simulink model "BD_PAR_saber_cosim"  (Simulink 4.1.1)
settings: Solver=ode1  SolverMode=SingleTasking  StartTime=0.0  StopTime=max(cyc_mph(:,1))  FixedStep=1  MaxStep=1  RelTol=1e-3  AbsTol=1e-3
undefined symbols (not defined in the file): cs_charge_deplete_bool, cs_electric_decel_spd, cs_electric_launch_spd_hi, cs_electric_launch_spd_lo, cs_hi_soc, cs_lo_soc, cs_off_trq_frac, cyc_mph, ess_on, ex_calc, fc_emis, fc_map_spd, fc_max_trq, fc_on, fc_spd_scale, fc_trq_scale, fc_tstat, fd_ratio, gb_dnshift_load, gb_dnshift_spd, gb_gears_num, gb_num_init, gb_ratio, gb_shift_delay, gb_upshift_load, gb_upshift_spd, mc_map_spd, mc_max_trq, mc_output_switch, mc_overtrq_factor, mc_spd_scale, mc_trq_scale, tc_mc_to_fc_ratio, time_step, tx_speed_dep, vc_clutch_bool, vc_fc_warm_tmp_frac, vc_idle_bool, vc_idle_spd, vc_launch_spd, wh_radius
libraries: lib_cosimulation x9, lib_outputs x7, lib_controls x6, lib_transmission x4, lib_wheel x2, simulink3 x2, lib_help x2, lib_interactive x1, lib_accessory x1, lib_drive_cycle x1, lib_exhaust x1, lib_fuel_converter x1
(part 1 of 2)
settings Model: LastModifiedBy=ssprik  SaveTime=off  SaveOutput=off  LimitDataPoints=off  UnconnectedLineMsg=none  RTWTemplateMakefile=grt_vc.tmf  ExtModeTrigMode=oneshot  ExtModeArmWhenConnect=off

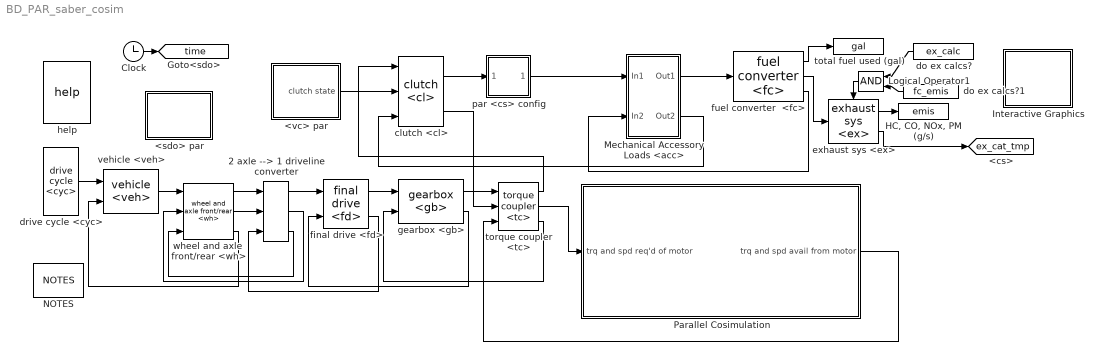
== system BD_PAR_saber_cosim ==
  2 axle --> 1 driveline converter : lib_wheel/2 axle --> 1 driveline converter
      settings: RTWFcnNameOpts=Auto  RTWFileNameOpts=Auto
  <sdo> par : Subsystem
      settings: RTWFcnNameOpts=Auto  RTWFileNameOpts=Auto
      mask Display: image(imread('bdi_sdo.jpg'))
  <vc> par : Subsystem
      settings: RTWFcnNameOpts=Auto  RTWFileNameOpts=Auto
      mask Display: image(imread('bdi_vc.jpg'))
  Clock : Clock
      settings: DisplayTime=off  Decimation=10
  "HC, CO, NOx, PM (g/s)" : ToWorkspace  VariableName=emis  SampleTime=0  SaveFormat=Array
  Interactive Graphics : Subsystem  BlockChoice=off
      link override off/Live Inputs/veh/roll res interactive: BlockChoice=roll res force req (N)
      settings: AttributesFormatString=%<BlockChoice>  TemplateBlock=lib_interactive/Interactive Graphics  MemberBlocks=off,on  RTWFcnNameOpts=Auto  RTWFileNameOpts=Auto
  Logical Operator1 : Logic  Orientation=left  Operator=AND  Inputs=2
  Mechanical Accessory Loads <acc> : Subsystem
      settings: RTWFcnNameOpts=Auto  RTWFileNameOpts=Auto
      mask Display: image(imread('bdi_acc_pic.bmp'))
  NOTES : lib_help/NOTES
  Parallel Cosimulation : Subsystem
      settings: RTWFcnNameOpts=Auto  RTWFileNameOpts=Auto
      mask Display: image(imread('par_cosim.bmp'))
  clutch <cl> : lib_transmission/clutch <cl>  slip_spd=vc_launch_spd  maxtrq=max(fc_max_trq)*fc_trq_scale
  do ex calcs? : Constant  Orientation=left  Value=ex_calc
  do ex calcs?1 : Constant  Orientation=left  Value=fc_emis
  drive cycle <cyc> : lib_drive_cycle/drive cycle <cyc>
  exhaust sys <ex> : lib_exhaust/exhaust sys <ex>
  final drive <fd> : lib_transmission/final drive <fd>
  fuel converter  <fc> : lib_fuel_converter/fuel converter  <fc>
      link override fuel use and EO emis Configurable Subsystem: BlockChoice=fuel use and EO emis
  gearbox <gb> : lib_transmission/gearbox <gb>
  help : lib_help/help
  par <cs> config : Subsystem  BlockChoice=electric assist control strategy <cs>
      settings: AttributesFormatString=%<BlockChoice>  TemplateBlock=lib_controls/par <cs> config  MemberBlocks=Adaptive control strategy <cs>,Fuzzy Logic control strategy <cs>,Fuzzy Logic control strategy with Emissions <cs>,electric assist control strategy <cs>,electric assist control strategy bal <cs>  RTWFcnNameOpts=Auto  RTWFileNameOpts=Auto
  torque coupler <tc> : lib_transmission/torque coupler <tc>
  total fuel used (gal) : ToWorkspace  VariableName=gal  SampleTime=0  SaveFormat=Array
  vehicle <veh> : lib_vehicle/vehicle <veh>
      link override record achieved force outputs/rolling resistance force: BlockChoice=force req'd to overcome rolling resistance (N)
      link override rolling resistance force: BlockChoice=force req'd to overcome rolling resistance (N)
      link override vehicle speed: BlockChoice=vehicle speed (m/s)
  wheel and axle  front/rear <wh> : lib_wheel/wheel and axle  front//rear <wh>
  tag scope: ex_cat_tmp=global, time=global
  wires:
  wheel and axle  front/rear <wh>/3 -> vehicle <veh>/2
  final drive <fd>/2 -> 2 axle --> 1 driveline converter/3
  final drive <fd>/1 -> gearbox <gb>/1
  drive cycle <cyc>/1 -> vehicle <veh>/1
  clutch <cl>/1 -> par <cs> config/1("trq and spd req'd into clutch (N*m, rad/s)")
  fuel converter  <fc>/2 -> exhaust sys <ex>/1
  do ex calcs?/1 -> Logical Operator1/1
  fuel converter  <fc>/1 -> total fuel used (gal)/1
  exhaust sys <ex>/1 -> "HC, CO, NOx, PM (g/s)"/1
  Logical Operator1/1 -> exhaust sys <ex>/Enable
  do ex calcs?1/1 -> Logical Operator1/2
  Clock/1 -> [time]
  gearbox <gb>/2 -> final drive <fd>/2
  torque coupler <tc>/3 -> gearbox <gb>/2
  torque coupler <tc>/1 -> clutch <cl>/1
  clutch <cl>/2 -> torque coupler <tc>/2
  gearbox <gb>/1 -> torque coupler <tc>/1
  <vc> par/1(clutch state) -> clutch <cl>/2
  torque coupler <tc>/2 -> Parallel Cosimulation/1(trq and spd req'd of motor)
  exhaust sys <ex>/2 -> [ex_cat_tmp]
  Parallel Cosimulation/1(trq and spd avail from motor) -> torque coupler <tc>/3
  par <cs> config/1("trq and spd req'd from engine (N*m, rad/s)") -> Mechanical Accessory Loads <acc>/1(In1)
  Mechanical Accessory Loads <acc>/1(Out1) -> fuel converter  <fc>/1
  fuel converter  <fc>/3 -> Mechanical Accessory Loads <acc>/2(In2)
  Mechanical Accessory Loads <acc>/2(Out2) -> clutch <cl>/3
  vehicle <veh>/1 -> wheel and axle  front/rear <wh>/1
  wheel and axle  front/rear <wh>/1 -> 2 axle --> 1 driveline converter/1
  wheel and axle  front/rear <wh>/2 -> 2 axle --> 1 driveline converter/2
  2 axle --> 1 driveline converter/1 -> final drive <fd>/1
  2 axle --> 1 driveline converter/2 -> wheel and axle  front/rear <wh>/2
  2 axle --> 1 driveline converter/3 -> wheel and axle  front/rear <wh>/3

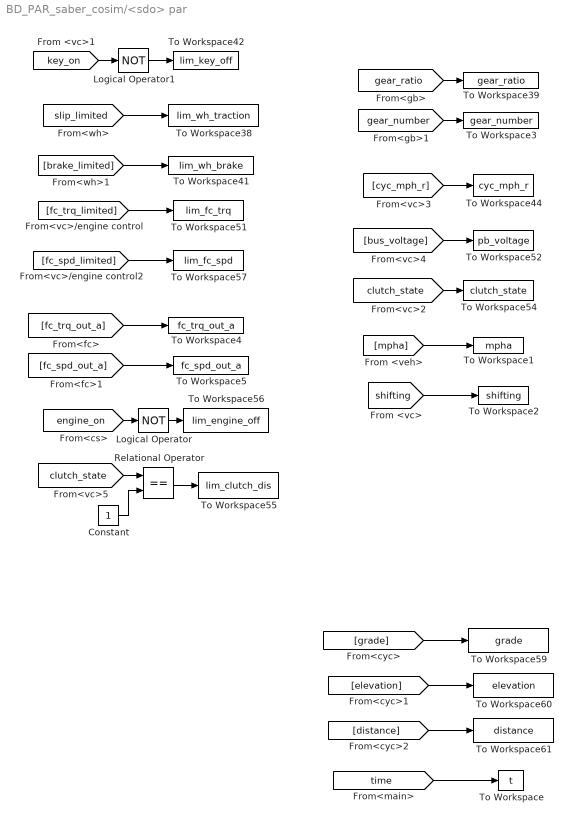
== system BD_PAR_saber_cosim/<sdo> par ==
  Constant : Constant  Value=1
  Logical Operator : Logic  Operator=NOT  Inputs=1
  Logical Operator1 : Logic  Operator=NOT  Inputs=1
  Relational Operator : RelationalOperator  Operator===
  To Workspace : ToWorkspace  VariableName=t  SampleTime=0  SaveFormat=Array
  To Workspace1 : ToWorkspace  VariableName=mpha  SampleTime=-1  SaveFormat=Array
  To Workspace2 : ToWorkspace  VariableName=shifting  SampleTime=-1  SaveFormat=Array
  To Workspace3 : ToWorkspace  VariableName=gear_number  SampleTime=-1  SaveFormat=Array
  To Workspace38 : ToWorkspace  VariableName=lim_wh_traction  SampleTime=-1  SaveFormat=Array
  To Workspace39 : ToWorkspace  VariableName=gear_ratio  SampleTime=-1  SaveFormat=Array
  To Workspace4 : ToWorkspace  VariableName=fc_trq_out_a  SampleTime=-1  SaveFormat=Array
  To Workspace41 : ToWorkspace  VariableName=lim_wh_brake  SampleTime=-1  SaveFormat=Array
  To Workspace42 : ToWorkspace  VariableName=lim_key_off  SampleTime=-1  SaveFormat=Array
  To Workspace44 : ToWorkspace  VariableName=cyc_mph_r  SampleTime=-1  SaveFormat=Array
  To Workspace5 : ToWorkspace  VariableName=fc_spd_out_a  SampleTime=-1  SaveFormat=Array
  To Workspace51 : ToWorkspace  VariableName=lim_fc_trq  SampleTime=-1  SaveFormat=Array
  To Workspace52 : ToWorkspace  VariableName=pb_voltage  SampleTime=-1  SaveFormat=Array
  To Workspace54 : ToWorkspace  VariableName=clutch_state  SampleTime=-1  SaveFormat=Array
  To Workspace55 : ToWorkspace  VariableName=lim_clutch_dis  SampleTime=-1  SaveFormat=Array
  To Workspace56 : ToWorkspace  VariableName=lim_engine_off  SampleTime=-1  SaveFormat=Array
  To Workspace57 : ToWorkspace  VariableName=lim_fc_spd  SampleTime=-1  SaveFormat=Array
  To Workspace59 : ToWorkspace  VariableName=grade  SampleTime=-1  SaveFormat=Array
  To Workspace60 : ToWorkspace  VariableName=elevation  SampleTime=-1  SaveFormat=Array
  To Workspace61 : ToWorkspace  VariableName=distance  SampleTime=-1  SaveFormat=Array
  wires:
  [time] -> To Workspace/1
  [fc_spd_out_a] -> To Workspace5/1
  [fc_trq_out_a] -> To Workspace4/1
  Relational Operator/1 -> To Workspace55/1
  Logical Operator/1 -> To Workspace56/1
  [engine_on] -> Logical Operator/1
  Constant/1 -> Relational Operator/2
  [clutch_state] -> Relational Operator/1
  [distance] -> To Workspace61/1
  [elevation] -> To Workspace60/1
  [grade] -> To Workspace59/1
  [brake_limited] -> To Workspace41/1
  [slip_limited] -> To Workspace38/1
  Logical Operator1/1 -> To Workspace42/1
  [key_on] -> Logical Operator1/1
  [shifting] -> To Workspace2/1
  [mpha] -> To Workspace1/1
  [clutch_state] -> To Workspace54/1
  [bus_voltage] -> To Workspace52/1
  [cyc_mph_r] -> To Workspace44/1
  [gear_ratio] -> To Workspace39/1
  [fc_spd_limited] -> To Workspace57/1
  [fc_trq_limited] -> To Workspace51/1
  [gear_number] -> To Workspace3/1

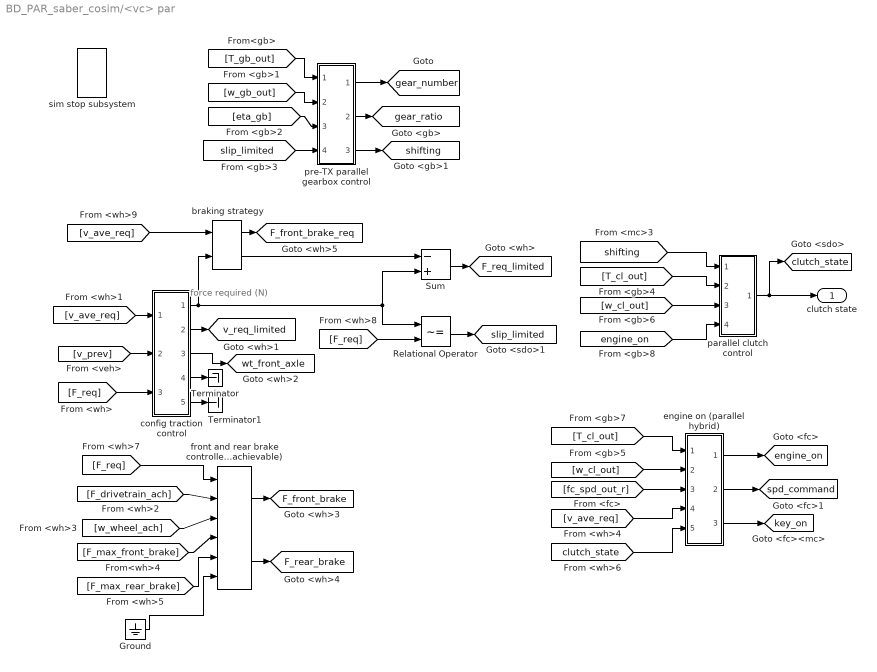
== system BD_PAR_saber_cosim/<vc> par ==
  note: force
      | required (N)
  Ground : Ground
  Relational Operator : RelationalOperator  Operator=~=
  Sum : Sum  Inputs=-+  SaturateOnIntegerOverflow=on
  Terminator : Terminator
  Terminator1 : Terminator
  braking strategy : lib_controls/SubSystem/braking strategy
      settings: RTWFcnNameOpts=Auto  RTWFileNameOpts=Auto
  config traction control : Subsystem  BlockChoice=traction control 2 axle
      settings: AttributesFormatString=%<BlockChoice>  TemplateBlock=lib_controls/SubSystem/config traction control  MemberBlocks=traction control 2 axle,traction control J2452 2 axle  RTWFcnNameOpts=Auto  RTWFileNameOpts=Auto
  engine on (parallel hybrid) : Subsystem
      settings: RTWFcnNameOpts=Auto  RTWFileNameOpts=Auto
  front and rear brake controller (achievable) : lib_controls/SubSystem/front and rear brake controller (achievable)
      settings: RTWFcnNameOpts=Auto  RTWFileNameOpts=Auto
  parallel clutch control : Subsystem
      settings: RTWFcnNameOpts=Auto  RTWFileNameOpts=Auto
  pre-TX parallel gearbox control : Subsystem
      settings: RTWFcnNameOpts=Auto  RTWFileNameOpts=Auto
  sim stop subsystem : lib_controls/SubSystem/sim stop subsystem
      settings: RTWFcnNameOpts=Auto  RTWFileNameOpts=Auto
  clutch state : Outport  Port=1
  tag scope: F_front_brake=global, F_front_brake_req=global, F_rear_brake=global, F_req_limited=global, clutch_state=global, engine_on=global, gear_number=global, gear_ratio=global, key_on=global, shifting=global, slip_limited=global, spd_command=global, v_req_limited=global, wt_front_axle=global
  wires:
  pre-TX parallel gearbox control/3("shifting, out") -> [shifting]
  pre-TX parallel gearbox control/2("gear ratio, out") -> [gear_ratio]
  pre-TX parallel gearbox control/1("gear number, out") -> [gear_number]
  [F_req] -> front and rear brake controller (achievable)/1
  front and rear brake controller (achievable)/2 -> [F_rear_brake]
  [F_max_rear_brake] -> front and rear brake controller (achievable)/5
  [F_max_front_brake] -> front and rear brake controller (achievable)/4
  [w_wheel_ach] -> front and rear brake controller (achievable)/3
  [F_drivetrain_ach] -> front and rear brake controller (achievable)/2
  front and rear brake controller (achievable)/1 -> [F_front_brake]
  [v_ave_req] -> braking strategy/1
  [v_ave_req] -> config traction control/1(time-average vehicle speed  req'd (m/s))
  [F_req] -> Relational Operator/2
  Relational Operator/1 -> [slip_limited]
  parallel clutch control/1(clutch state) -> clutch state/1, [clutch_state]
  [engine_on] -> parallel clutch control/4(engine on)
  [T_cl_out] -> parallel clutch control/2(gb_trq_in_r)
  [w_cl_out] -> parallel clutch control/3(gb_spd_in_r)
  [shifting] -> parallel clutch control/1(shifting)
  Sum/1 -> [F_req_limited]
  [F_req] -> config traction control/3(total tractive force req'd (N))
  config traction control/2(req'd speed (m/s)) -> [v_req_limited]
  [v_prev] -> config traction control/2(vehicle speed at beginning of time  step (m/s))
  braking strategy/1 -> [F_front_brake_req]
  config traction control/1(req'd force (N)) -> Relational Operator/1, Sum/2, braking strategy/2
  braking strategy/2 -> Sum/1
  [clutch_state] -> engine on (parallel hybrid)/5(clutch state)
  engine on (parallel hybrid)/1(engine on) -> [engine_on]
  [T_cl_out] -> engine on (parallel hybrid)/1(trq req'd out of clutch (N*m))
  [w_cl_out] -> engine on (parallel hybrid)/2(spd req'd out of clutch (N*m)1)
  [v_ave_req] -> engine on (parallel hybrid)/4(v_ave_req)
  engine on (parallel hybrid)/2(spd command  (rad/s)) -> [spd_command]
  [fc_spd_out_r] -> engine on (parallel hybrid)/3(fc_spd_out_r)
  engine on (parallel hybrid)/3(key on) -> [key_on]
  [eta_gb] -> pre-TX parallel gearbox control/3(prev. Pout/Pin)
  [w_gb_out] -> pre-TX parallel gearbox control/2(gb_spd_out_r)
  [T_gb_out] -> pre-TX parallel gearbox control/1(gb_trq_out_r)
  [slip_limited] -> pre-TX parallel gearbox control/4(tires are at traction limit)
  config traction control/3(weight on front axle (N)) -> [wt_front_axle]
  config traction control/4(weight on rear axle (N)) -> Terminator/1
  config traction control/5(front/total  traction ratio) -> Terminator1/1
  Ground/1 -> front and rear brake controller (achievable)/6

== system BD_PAR_saber_cosim/Interactive Graphics ==
  off : lib_interactive/off  Tag=Altia_off  Orientation=up

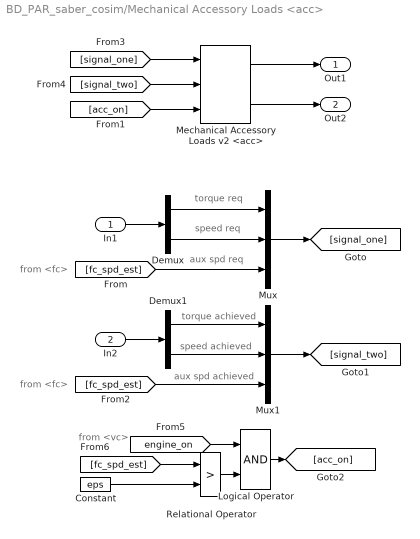
== system BD_PAR_saber_cosim/Mechanical Accessory Loads <acc> ==
  note: from <vc>
  note: aux spd achieved
  note: speed achieved
  note: torque achieved
  note: aux spd req
  note: speed req
  note: torque req
  note: from <fc>
  note: from <fc>
  In1 : Inport  Port=1  LatchInput=off
  In2 : Inport  Port=2  LatchInput=off
  Constant : Constant  Value=eps
  Demux : Demux  Outputs=2  BusSelectionMode=off
  Demux1 : Demux  Outputs=2  BusSelectionMode=off
  Logical Operator : Logic  Operator=AND  Inputs=2
  Mechanical Accessory Loads v2 <acc> : lib_accessory/Mechanical Accessory Loads v2 <acc>  load_on=not(ess_on)*1  acc_max_spd=inf  acc_min_spd=(vc_idle_spd*vc_idle_bool)+eps  ic_mech_trq=0  ic_mech_pwr=0
      link override backward model/mechanical accessories (Nm): BlockChoice=Mechanical Accessories: Speed Dependant and Variable Electrical
      link override estimated mechanical torque/mechanical accessories (Nm): BlockChoice=Mechanical Accessories: Const Mech Var Elect
  Mux : Mux  Inputs=3
  Mux1 : Mux  Inputs=3
  Relational Operator : RelationalOperator  Operator=>
  Out1 : Outport  Port=1
  Out2 : Outport  Port=2
  wires:
  Logical Operator/1 -> [acc_on]
  Relational Operator/1 -> Logical Operator/2
  [engine_on] -> Logical Operator/1
  Constant/1 -> Relational Operator/2
  [fc_spd_est] -> Relational Operator/1
  [fc_spd_est] -> Mux1/3
  Demux1/2 -> Mux1/2
  Demux1/1 -> Mux1/1
  In2/1 -> Demux1/1
  Mux1/1 -> [signal_two]
  [fc_spd_est] -> Mux/3
  Demux/2 -> Mux/2
  Demux/1 -> Mux/1
  In1/1 -> Demux/1
  Mux/1 -> [signal_one]
  [acc_on] -> Mechanical Accessory Loads v2 <acc>/3
  [signal_two] -> Mechanical Accessory Loads v2 <acc>/2
  Mechanical Accessory Loads v2 <acc>/2 -> Out2/1
  Mechanical Accessory Loads v2 <acc>/1 -> Out1/1
  [signal_one] -> Mechanical Accessory Loads v2 <acc>/1

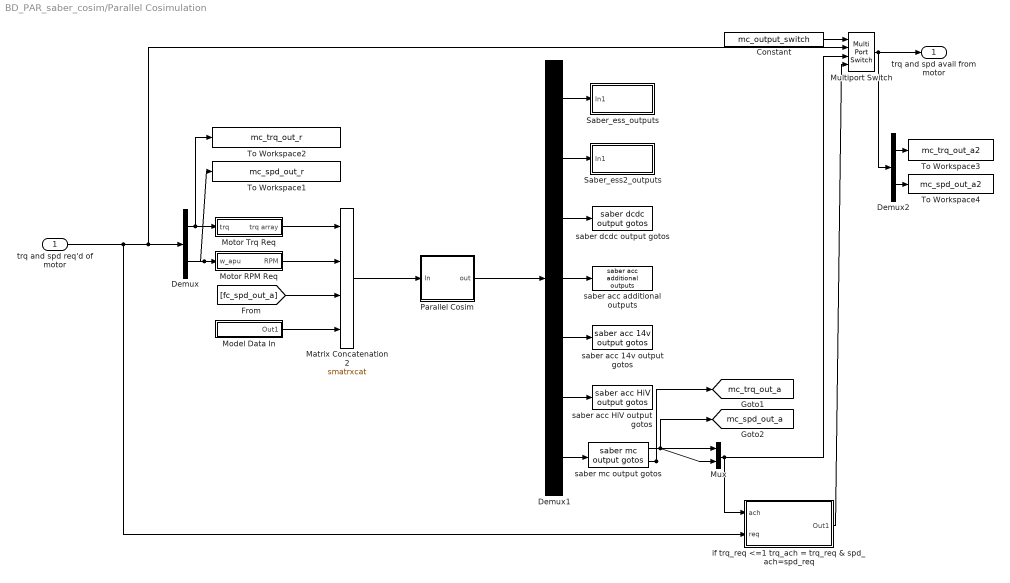
== system BD_PAR_saber_cosim/Parallel Cosimulation ==
  trq and spd req'd of motor : Inport  Port=1  LatchInput=off
  Constant : Constant  Value=mc_output_switch
  Demux : Demux  Outputs=2  BusSelectionMode=off
  Demux1 : Demux  Outputs=[4 4 2 2 30 12 4]  BusSelectionMode=off
  Demux2 : Demux  Outputs=2  BusSelectionMode=off
  Matrix Concatenation2 : S-Function  FunctionName=smatrxcat  Parameters=numInports,catMethod  PortCounts=[]  SFunctionModules=''  mask(Matrix Concatenation){numInports=4, catMethod=Horizontal}
      mask prompts: numInports "Number of inputs:"; catMethod "Concatenation method:"
      mask help: Perform horizontal or vertical concatenation. 1-D vector input signals are treated as column vectors, i.e., [Mx1] matrices. The output is always a matrix.
      mask init:
      | xy = matrxcatmask('icon');
      mask StyleString: edit,popup(Horizontal|Vertical)
      mask Display:
      | plot(xy.x,xy.y);
      | text(0.15,0.86,xy.label);
  Model Data In : Subsystem
      settings: RTWFcnNameOpts=Auto  RTWFileNameOpts=Auto
      mask Display: disp('Parallel')
  Motor RPM Req : Subsystem
      settings: RTWFcnNameOpts=Auto  RTWFileNameOpts=Auto
  Motor Trq Req : Subsystem
      settings: RTWFcnNameOpts=Auto  RTWFileNameOpts=Auto
  Multiport Switch : MultiPortSwitch  Inputs=3
  Mux : Mux  Inputs=2
  Parallel Cosim : Subsystem  BlockChoice=Par Saber Text File Exchange
      settings: AttributesFormatString=%<BlockChoice>  TemplateBlock=lib_cosimulation/Parallel Cosim  MemberBlocks=Par Saber Text File Exchange  RTWFcnNameOpts=Auto  RTWFileNameOpts=Auto
  Saber_ess2_outputs : Subsystem  BlockChoice=Saber_pb2
      settings: AttributesFormatString=%<BlockChoice>  TemplateBlock=lib_outputs/Saber_ess2_outputs  MemberBlocks=Saber_pb2,Saber_rint2  RTWFcnNameOpts=Auto  RTWFileNameOpts=Auto
  Saber_ess_outputs : Subsystem  BlockChoice=Saber_pb
      settings: AttributesFormatString=%<BlockChoice>  TemplateBlock=lib_outputs/Saber_ess_outputs  MemberBlocks=Saber_pb,Saber_rint  RTWFcnNameOpts=Auto  RTWFileNameOpts=Auto
  To Workspace1 : ToWorkspace  VariableName=mc_spd_out_r  SampleTime=-1  SaveFormat=Array
  To Workspace2 : ToWorkspace  VariableName=mc_trq_out_r  SampleTime=-1  SaveFormat=Array
  To Workspace3 : ToWorkspace  VariableName=mc_trq_out_a2  SampleTime=-1  SaveFormat=Array
  To Workspace4 : ToWorkspace  VariableName=mc_spd_out_a2  SampleTime=-1  SaveFormat=Array
  if trq_req <=1 trq_ach = trq_req & spd_ach=spd_req : Subsystem
      settings: RTWFcnNameOpts=Auto  RTWFileNameOpts=Auto
  saber acc 14v output gotos : lib_outputs/saber acc 14v output gotos
      settings: RTWFcnNameOpts=Auto  RTWFileNameOpts=Auto
  saber acc HiV output gotos : lib_outputs/saber acc HiV output gotos
      settings: RTWFcnNameOpts=Auto  RTWFileNameOpts=Auto
  saber acc additional outputs : lib_outputs/saber acc additional outputs
      settings: RTWFcnNameOpts=Auto  RTWFileNameOpts=Auto
  saber dcdc output gotos : lib_outputs/saber dcdc output gotos
      settings: RTWFcnNameOpts=Auto  RTWFileNameOpts=Auto
  saber mc output gotos : lib_outputs/saber mc output gotos
      settings: RTWFcnNameOpts=Auto  RTWFileNameOpts=Auto
  trq and spd avail from motor : Outport  Port=1
  tag scope: mc_spd_out_a=global, mc_trq_out_a=global
  wires:
  trq and spd req'd of motor/1 -> if trq_req <=1 trq_ach = trq_req & spd_ach=spd_req/2(req), Demux/1, Multiport Switch/2
  Matrix Concatenation2/1 -> Parallel Cosim/1(In)
  Demux/1 -> To Workspace2/1, Motor Trq Req/1(trq)
  Demux/2 -> To Workspace1/1, Motor RPM Req/1(w_apu)
  Motor Trq Req/1(trq array) -> Matrix Concatenation2/1
  Motor RPM Req/1(RPM) -> Matrix Concatenation2/2
  Parallel Cosim/1(out) -> Demux1/1
  Demux1/3 -> saber dcdc output gotos/1
  saber mc output gotos/2 -> [mc_trq_out_a], Mux/1
  Demux1/2 -> Saber_ess2_outputs/1(In1)
  Demux1/1 -> Saber_ess_outputs/1(In1)
  saber mc output gotos/1 -> Mux/2, [mc_spd_out_a]
  [fc_spd_out_a] -> Matrix Concatenation2/3
  Model Data In/1(Out1) -> Matrix Concatenation2/4
  Mux/1 -> if trq_req <=1 trq_ach = trq_req & spd_ach=spd_req/1(ach), Multiport Switch/3
  Demux2/1 -> To Workspace3/1
  Demux2/2 -> To Workspace4/1
  Multiport Switch/1 -> trq and spd avail from motor/1, Demux2/1
  Constant/1 -> Multiport Switch/1
  if trq_req <=1 trq_ach = trq_req & spd_ach=spd_req/1(Out1) -> Multiport Switch/4
  Demux1/5 -> saber acc 14v output gotos/1
  Demux1/6 -> saber acc HiV output gotos/1
  Demux1/7 -> saber mc output gotos/1
  Demux1/4 -> saber acc additional outputs/1

== system BD_PAR_saber_cosim/par <cs> config ==
  "trq and spd req'd into clutch (N*m, rad/s)" : Inport  Port=1  LatchInput=off
  electric assist control strategy <cs> : lib_controls/electric assist control strategy <cs>
  "trq and spd req'd from engine (N*m, rad/s)" : Outport  Port=1
  wires:
  "trq and spd req'd into clutch (N*m, rad/s)"/1 -> electric assist control strategy <cs>/1
  electric assist control strategy <cs>/1 -> "trq and spd req'd from engine (N*m, rad/s)"/1

== system BD_PAR_saber_cosim/<vc> par/config traction control ==
  time-average vehicle speed  req'd (m/s) : Inport  Port=1  LatchInput=off
  vehicle speed at beginning of time  step (m/s) : Inport  Port=2  LatchInput=off
  total tractive force req'd (N) : Inport  Port=3  LatchInput=off
  traction control 2 axle : lib_controls/SubSystem/traction control 2 axle
      settings: RTWFcnNameOpts=Auto  RTWFileNameOpts=Auto
  req'd force (N) : Outport  Port=1
  req'd speed (m/s) : Outport  Port=2
  weight on front axle (N) : Outport  Port=3
  weight on rear axle (N) : Outport  Port=4
  front/total  traction ratio : Outport  Port=5
  wires:
  time-average vehicle speed  req'd (m/s)/1 -> traction control 2 axle/1
  vehicle speed at beginning of time  step (m/s)/1 -> traction control 2 axle/2
  total tractive force req'd (N)/1 -> traction control 2 axle/3
  traction control 2 axle/1 -> req'd force (N)/1
  traction control 2 axle/2 -> req'd speed (m/s)/1
  traction control 2 axle/3 -> weight on front axle (N)/1
  traction control 2 axle/4 -> weight on rear axle (N)/1
  traction control 2 axle/5 -> front/total  traction ratio/1

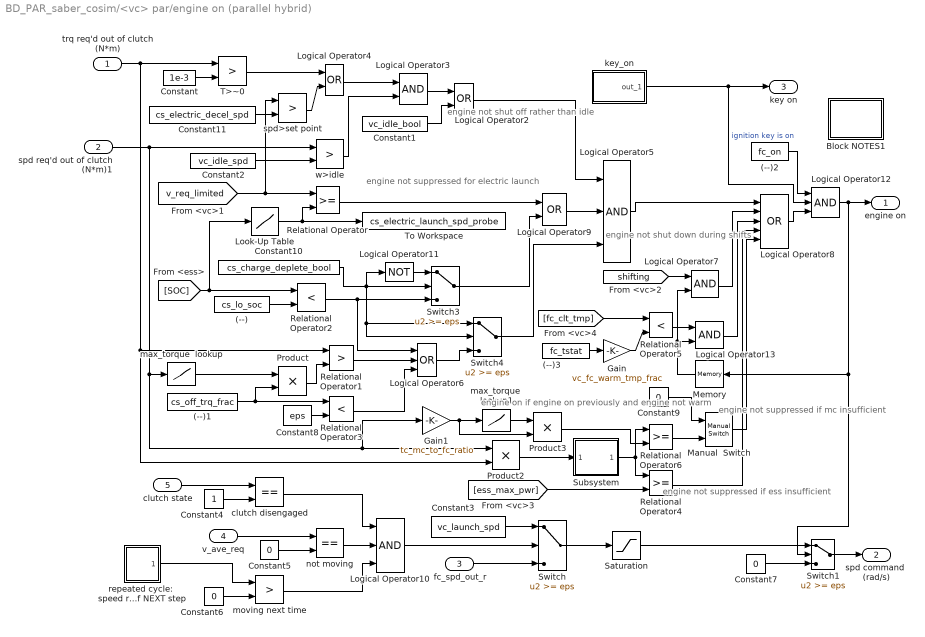
== system BD_PAR_saber_cosim/<vc> par/engine on (parallel hybrid) ==
  note: engine not suppressed
      | if mc insufficient
  note: engine not shut
      | down during shifts
  note: engine on if engine on
      | previously and engine
      | not warm
  note: engine not shut off
      |  rather than idle
  note: engine not
      | suppressed for
      | electric launch
  note: engine not suppressed if
      | ess insufficient
  trq req'd out of clutch (N*m) : Inport  Port=1  LatchInput=off
  spd req'd out of clutch (N*m)1 : Inport  Port=2  LatchInput=off
  fc_spd_out_r : Inport  Port=3  LatchInput=off
  v_ave_req : Inport  Port=4  LatchInput=off
  clutch state : Inport  Port=5  LatchInput=off
  (--) : Constant  Value=cs_lo_soc
  (--)1 : Constant  Value=cs_off_trq_frac
  (--)2 : Constant  Value=fc_on
  (--)3 : Constant  Value=fc_tstat
  Block NOTES1 : Subsystem
      settings: RTWFcnNameOpts=Auto  RTWFileNameOpts=Auto
      mask Display: disp('Block\nNOTES')
  Constant : Constant  Value=1e-3
  Constant1 : Constant  Value=vc_idle_bool
  Constant10 : Constant  Value=cs_charge_deplete_bool
  Constant11 : Constant  Value=cs_electric_decel_spd
  Constant2 : Constant  Value=vc_idle_spd
  Constant3 : Constant  Value=vc_launch_spd
  Constant4 : Constant  Value=1
  Constant{5..7,9} (4 alike) : Constant  Value=0
  Constant8 : Constant  Value=eps
  Gain : Gain  Gain=vc_fc_warm_tmp_frac  Multiplication=Element-wise(K.*u)  SaturateOnIntegerOverflow=on
  Gain1 : Gain  Gain=tc_mc_to_fc_ratio  Multiplication=Element-wise(K.*u)  SaturateOnIntegerOverflow=on
  Logical Operator10 : Logic  Operator=AND  Inputs=3
  Logical Operator11 : Logic  Operator=NOT  Inputs=1
  Logical Operator12 : Logic  Operator=AND  Inputs=3
  Logical Operator13 : Logic  Operator=AND  Inputs=2
  Logical Operator2 : Logic  Operator=OR  Inputs=2
  Logical Operator3 : Logic  Operator=AND  Inputs=2
  Logical Operator4 : Logic  Operator=OR  Inputs=2
  Logical Operator5 : Logic  Operator=AND  Inputs=3
  Logical Operator6 : Logic  Operator=OR  Inputs=3
  Logical Operator7 : Logic  Operator=AND  Inputs=2
  Logical Operator8 : Logic  Operator=OR  Inputs=5
  Logical Operator9 : Logic  Operator=OR  Inputs=2
  Look-Up Table : Lookup  InputValues=[cs_lo_soc cs_hi_soc cs_hi_soc+eps]  OutputValues=[cs_electric_launch_spd_lo cs_electric_launch_spd_hi cs_electric_launch_spd_hi]
  Manual  Switch : simulink3/Nonlinear/Manual Switch  sw=1  action=0
  Memory : Memory  Orientation=left  X0=cyc_mph(1,2)>0  InheritSampleTime=off
      settings: RTWStateStorageClass=Auto
  Product : Product  Inputs=2  Multiplication=Element-wise(.*)  SaturateOnIntegerOverflow=on
  Product2 : Product  Inputs=2  Multiplication=Element-wise(.*)  SaturateOnIntegerOverflow=on
  Product3 : Product  Inputs=2  Multiplication=Element-wise(.*)  SaturateOnIntegerOverflow=on
  Relational Operator : RelationalOperator  Operator=>=
  Relational Operator1 : RelationalOperator  Operator=>
  Relational Operator2 : RelationalOperator  Operator=<
  Relational Operator3 : RelationalOperator  Operator=<
  Relational Operator4 : RelationalOperator  Operator=>=
  Relational Operator5 : RelationalOperator  Operator=<
  Relational Operator6 : RelationalOperator  Operator=>=
  Saturation : Saturate  UpperLimit=max(fc_map_spd)*fc_spd_scale  LowerLimit=vc_idle_spd*vc_idle_bool  LinearizeAsGain=on
  Subsystem : Subsystem  mask(Running Average){n=3}
      mask prompts: n "Averaging Time Steps (#)"
      mask help: Running Average
      settings: RTWFcnNameOpts=Auto  RTWFileNameOpts=Auto
      mask Help: Output is the average of the last (Averaging Time) seconds of input.
      mask Display: disp('Running\nAverage')
  Switch{,1,3..4} (4 alike) : Switch  Threshold=eps
  T>~0 : RelationalOperator  Operator=>
  To Workspace : ToWorkspace  VariableName=cs_electric_launch_spd_probe  SampleTime=-1  SaveFormat=Array
  clutch disengaged : RelationalOperator  Operator===
  key_on : Subsystem  mask(Repeating table){@1=vc_key_on(:,1), @2=vc_key_on(:,2)}
      mask prompts: @1 "Time values:"; @2 "Output values:"
      mask help:
      | Repeating table.
      | Enter values of time and output for first cycle.
      mask init:
      | period = max(@1); t = @1; y = @2;
      settings: RTWFcnNameOpts=Auto  RTWFileNameOpts=Auto
      mask Help: Repeats cycle given in table. Time values should be monotonically increasing.
  max_torque  lookup : Lookup  InputValues=fc_map_spd*fc_spd_scale  OutputValues=fc_max_trq*fc_trq_scale
  max_torque  lookup1 : Lookup  InputValues=mc_map_spd*mc_spd_scale  OutputValues=mc_max_trq*mc_trq_scale*mc_overtrq_factor
  moving next time : RelationalOperator  Operator=>
  not moving : RelationalOperator  Operator===
  repeated cycle:  speed required at end of NEXT step : Subsystem  mask(Forward looking repeating table){t=cyc_mph(:,1), y=cyc_mph(:,2)}
      mask prompts: t "Time values:"; y "Output values:"
      mask help:
      | Forward looking repeating table.
      | Enter values of time and output for first cycle.
      mask init:
      | period = max(t);
      settings: RTWFcnNameOpts=Auto  RTWFileNameOpts=Auto
      mask Help: Repeats cycle given in table with a one time step forward offset. Time values should be monotonically increasing.
  spd>set point : RelationalOperator  Operator=>
  w>idle : RelationalOperator  Operator=>
  engine on : Outport  Port=1
  spd command  (rad/s) : Outport  Port=2
  key on : Outport  Port=3
  wires:
  Subsystem/1(out_1) -> Relational Operator6/1, Relational Operator4/1
  Product3/1 -> Relational Operator6/2
  [ess_max_pwr] -> Relational Operator4/2
  [v_req_limited] -> spd>set point/1, Relational Operator/1
  T>~0/1 -> Logical Operator4/1
  Logical Operator4/1 -> Logical Operator3/1
  spd>set point/1 -> Logical Operator4/2
  Constant11/1 -> spd>set point/2
  spd req'd out of clutch (N*m)1/1 -> w>idle/1, Gain1/1, Product2/1, max_torque  lookup/1
  w>idle/1 -> Logical Operator3/2
  Constant2/1 -> w>idle/2
  Constant9/1 -> Manual  Switch/1
  Manual  Switch/1 -> Logical Operator8/5
  Relational Operator6/1 -> Manual  Switch/2
  Gain1/1 -> Product3/2, max_torque  lookup1/1
  max_torque  lookup1/1 -> Product3/1
  Relational Operator3/1 -> Logical Operator6/3
  Product2/1 -> Subsystem/1(in_1)
  Constant4/1 -> clutch disengaged/2
  clutch state/1 -> clutch disengaged/1
  Constant5/1 -> not moving/2
  v_ave_req/1 -> not moving/1
  not moving/1 -> Logical Operator10/2
  moving next time/1 -> Logical Operator10/3
  clutch disengaged/1 -> Logical Operator10/1
  Constant6/1 -> moving next time/2
  repeated cycle:  speed required at end of NEXT step/1(out_1) -> moving next time/1
  Constant7/1 -> Switch1/3
  Switch1/1 -> spd command  (rad/s)/1
  Saturation/1 -> Switch1/1
  fc_spd_out_r/1 -> Switch/3
  Logical Operator10/1 -> Switch/2
  Switch/1 -> Saturation/1
  Constant3/1 -> Switch/1
  Relational Operator4/1 -> Logical Operator8/4
  (--)/1 -> Relational Operator2/2
  [SOC] -> Look-Up Table/1, Relational Operator2/1
  Logical Operator11/1 -> Switch3/1
  Relational Operator2/1 -> Logical Operator6/1, Switch3/3
  Constant10/1 -> Logical Operator11/1, Switch3/2, Switch4/2, Switch4/1
  Look-Up Table/1 -> To Workspace/1, Relational Operator/2
  Relational Operator/1 -> Logical Operator9/1
  Switch4/1 -> Logical Operator5/3
  Logical Operator9/1 -> Logical Operator5/2
  Logical Operator2/1 -> Logical Operator5/1
  key_on/1(out_1) -> Logical Operator12/2, key on/1  "ignition key is on"
  Logical Operator8/1 -> Logical Operator12/3
  (--)3/1 -> Gain/1
  Gain/1 -> Relational Operator5/2
  Logical Operator13/1 -> Logical Operator8/3
  [fc_clt_tmp] -> Relational Operator5/1
  Relational Operator5/1 -> Logical Operator13/1
  Memory/1 -> Logical Operator13/2, Logical Operator7/2
  Relational Operator1/1 -> Logical Operator6/2
  Logical Operator5/1 -> Logical Operator8/1
  Logical Operator3/1 -> Logical Operator2/1
  Constant1/1 -> Logical Operator2/2
  trq req'd out of clutch (N*m)/1 -> Relational Operator1/1, Product2/2, T>~0/1
  Logical Operator7/1 -> Logical Operator8/2
  [shifting] -> Logical Operator7/1
  Constant/1 -> T>~0/2
  Switch3/1 -> Logical Operator9/2
  Logical Operator6/1 -> Switch4/3
  Constant8/1 -> Relational Operator3/2
  (--)1/1 -> Relational Operator3/1, Product/2
  Product/1 -> Relational Operator1/2
  max_torque  lookup/1 -> Product/1
  (--)2/1 -> Logical Operator12/1
  Logical Operator12/1 -> engine on/1, Memory/1, Switch1/2

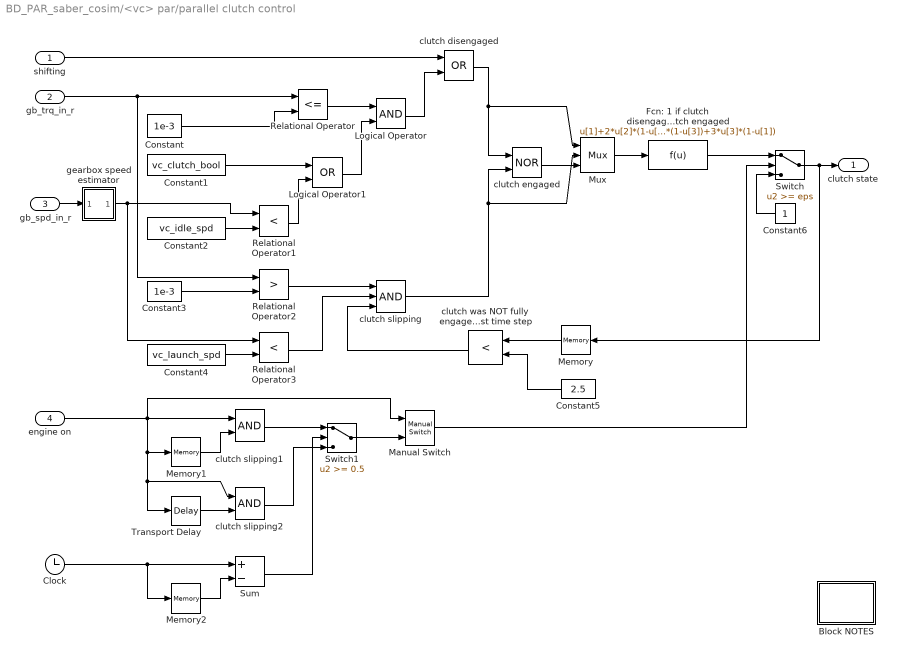
== system BD_PAR_saber_cosim/<vc> par/parallel clutch control ==
  shifting : Inport  Port=1  LatchInput=off
  gb_trq_in_r : Inport  Port=2  LatchInput=off
  gb_spd_in_r : Inport  Port=3  LatchInput=off
  engine on : Inport  Port=4  LatchInput=off
  Block NOTES : Subsystem
      settings: RTWFcnNameOpts=Auto  RTWFileNameOpts=Auto
      mask Display: disp('Block\nNOTES')
  Clock : Clock
      settings: DisplayTime=off  Decimation=10
  Constant : Constant  Value=1e-3
  Constant1 : Constant  Value=vc_clutch_bool
  Constant2 : Constant  Value=vc_idle_spd
  Constant3 : Constant  Value=1e-3
  Constant4 : Constant  Value=vc_launch_spd
  Constant5 : Constant  Orientation=left  Value=2.5
  Constant6 : Constant  Orientation=left  Value=1
  Fcn: 1 if clutch disengaged 2 if clutch slipping 3 if clutch engaged : Fcn  Expr=u[1]+2*u[2]*(1-u[1])*(1-u[3])+3*u[3]*(1-u[1])
  Logical Operator : Logic  Operator=AND  Inputs=2
  Logical Operator1 : Logic  Operator=OR  Inputs=2
  Manual Switch : simulink3/Nonlinear/Manual Switch  sw=1  action=0
  Memory : Memory  Orientation=left  X0=1+(2*(cyc_mph(1,2)>0))  InheritSampleTime=off
      settings: RTWStateStorageClass=Auto
  Memory1 : Memory  X0=cyc_mph(1,2)>0  InheritSampleTime=off
      settings: RTWStateStorageClass=Auto
  Memory2 : Memory  X0=-1  InheritSampleTime=off
      settings: RTWStateStorageClass=Auto
  Mux : Mux  Inputs=3
      settings: DisplayOption=none
  Relational Operator : RelationalOperator  Operator=<=
  Relational Operator1 : RelationalOperator  Operator=<
  Relational Operator2 : RelationalOperator  Operator=>
  Relational Operator3 : RelationalOperator  Operator=<
  Sum : Sum  Inputs=+-  SaturateOnIntegerOverflow=on
  Switch : Switch  Threshold=eps
  Switch1 : Switch  Threshold=0.5
  Transport Delay : TransportDelay  DelayTime=0.2  InitialInput=0  BufferSize=1024  PadeOrder=0
  clutch disengaged : Logic  Operator=OR  Inputs=2
  clutch engaged : Logic  Operator=NOR  Inputs=2
  clutch slipping : Logic  Operator=AND  Inputs=3
  clutch slipping1 : Logic  Operator=AND  Inputs=2
  clutch slipping2 : Logic  Operator=AND  Inputs=2
  clutch was NOT fully engaged during last time step : RelationalOperator  Orientation=left  Operator=<
  gearbox speed estimator : Subsystem
      settings: RTWFcnNameOpts=Auto  RTWFileNameOpts=Auto
  clutch state : Outport  Port=1
  wires:
  Switch/1 -> Memory/1, clutch state/1
  Fcn: 1 if clutch disengaged 2 if clutch slipping 3 if clutch engaged/1 -> Switch/1
  Manual Switch/1 -> Switch/2
  Switch1/1 -> Manual Switch/2
  gearbox speed estimator/1(Out1) -> Relational Operator3/1, Relational Operator1/1
  gb_spd_in_r/1 -> gearbox speed estimator/1(gb_spd_in_r if no gear change)
  Sum/1 -> Switch1/2
  Memory2/1 -> Sum/2
  Clock/1 -> Memory2/1, Sum/1
  clutch slipping2/1 -> Switch1/3
  Transport Delay/1 -> clutch slipping2/2
  clutch slipping1/1 -> Switch1/1
  Memory1/1 -> clutch slipping1/2
  engine on/1 -> Manual Switch/1, clutch slipping2/1, Transport Delay/1, Memory1/1, clutch slipping1/1
  Relational Operator1/1 -> Logical Operator1/2
  Constant2/1 -> Relational Operator1/2
  Mux/1 -> Fcn: 1 if clutch disengaged 2 if clutch slipping 3 if clutch engaged/1
  clutch engaged/1 -> Mux/3
  clutch disengaged/1 -> clutch engaged/1, Mux/1
  Constant3/1 -> Relational Operator2/2
  Relational Operator2/1 -> clutch slipping/1
  clutch slipping/1 -> clutch engaged/2, Mux/2
  Constant4/1 -> Relational Operator3/2
  Relational Operator3/1 -> clutch slipping/2
  Memory/1 -> clutch was NOT fully engaged during last time step/1
  Constant5/1 -> clutch was NOT fully engaged during last time step/2
  clutch was NOT fully engaged during last time step/1 -> clutch slipping/3
  Constant1/1 -> Logical Operator1/1
  Constant/1 -> Relational Operator/2
  Relational Operator/1 -> Logical Operator/1
  Logical Operator1/1 -> Logical Operator/2
  gb_trq_in_r/1 -> Relational Operator2/1, Relational Operator/1
  Logical Operator/1 -> clutch disengaged/2
  shifting/1 -> clutch disengaged/1
  Constant6/1 -> Switch/3

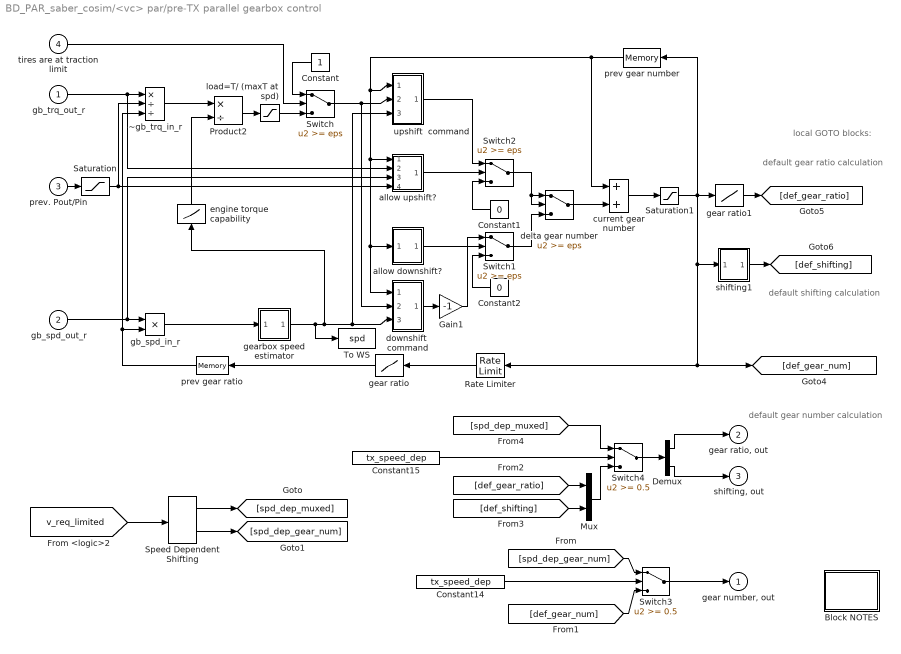
== system BD_PAR_saber_cosim/<vc> par/pre-TX parallel gearbox control ==
  note: local GOTO blocks:
  note: default gear ratio
      | calculation
  note: default shifting
      | calculation
  note: default gear number
      | calculation
  gb_trq_out_r : Inport  Port=1  LatchInput=off
  gb_spd_out_r : Inport  Port=2  LatchInput=off
  prev. Pout/Pin : Inport  Port=3  LatchInput=off
  tires are at traction limit : Inport  Port=4  LatchInput=off
  Block NOTES : Subsystem
      settings: RTWFcnNameOpts=Auto  RTWFileNameOpts=Auto
      mask Display: disp('Block\nNOTES')
  Constant : Constant  Orientation=left  Value=1
  Constant1 : Constant  Orientation=left  Value=0
  Constant14 : Constant  Value=tx_speed_dep
  Constant15 : Constant  Value=tx_speed_dep
  Constant2 : Constant  Orientation=left  Value=0
  Demux : Demux  Outputs=2  BusSelectionMode=off
  Gain1 : Gain  Gain=-1  Multiplication=Element-wise(K.*u)  SaturateOnIntegerOverflow=on
  Mux : Mux  Inputs=2
  Product2 : Product  Inputs=*/  Multiplication=Element-wise(.*)  SaturateOnIntegerOverflow=on
  Rate Limiter : RateLimiter  Orientation=left  RisingSlewLimit=1/(gb_shift_delay+eps)  FallingSlewLimit=-1/(gb_shift_delay+eps)
  Saturation : Saturate  UpperLimit=1  LowerLimit=0.2  LinearizeAsGain=on
  Saturation1 : Saturate  UpperLimit=gb_gears_num  LowerLimit=1  LinearizeAsGain=on
  Speed Dependent Shifting : lib_controls/SubSystem/Speed Dependent Shifting
      settings: RTWFcnNameOpts=Auto  RTWFileNameOpts=Auto
  Switch : Switch  Threshold=eps
  Switch1 : Switch  Threshold=eps
  Switch2 : Switch  Threshold=eps
  Switch3 : Switch  Threshold=0.5
  Switch4 : Switch  Threshold=0.5
  To WS : ToWorkspace  VariableName=spd  SampleTime=-1  SaveFormat=Array
  allow downshift? : Subsystem
      settings: RTWFcnNameOpts=Auto  RTWFileNameOpts=Auto
  allow upshift? : Subsystem
      settings: RTWFcnNameOpts=Auto  RTWFileNameOpts=Auto
  current gear number : Sum  Inputs=++  SaturateOnIntegerOverflow=on
  delta gear number : Switch  Threshold=eps
  downshift  command : Subsystem
      settings: RTWFcnNameOpts=Auto  RTWFileNameOpts=Auto
  engine torque capability : Lookup  Orientation=up  InputValues=fc_map_spd*fc_spd_scale  OutputValues=fc_max_trq*fc_trq_scale+eps
  gb_spd_in_r : Product  Inputs=2  Multiplication=Element-wise(.*)  SaturateOnIntegerOverflow=on
  gear ratio : Lookup  Orientation=left  InputValues=[1:length(gb_ratio)]  OutputValues=gb_ratio
  gear ratio1 : Lookup  InputValues=[1:length(gb_ratio)]  OutputValues=gb_ratio
  gearbox speed estimator : Subsystem
      settings: RTWFcnNameOpts=Auto  RTWFileNameOpts=Auto
  load=T/ (maxT at spd) : Saturate  UpperLimit=1  LowerLimit=0  LinearizeAsGain=on
  prev gear number : Memory  Orientation=left  X0=gb_num_init  InheritSampleTime=off
      settings: RTWStateStorageClass=Auto
  prev gear ratio : Memory  Orientation=left  X0=gb_ratio(gb_num_init)  InheritSampleTime=off
      settings: RTWStateStorageClass=Auto
  shifting1 : Subsystem
      settings: RTWFcnNameOpts=Auto  RTWFileNameOpts=Auto
  upshift  command : Subsystem
      settings: RTWFcnNameOpts=Auto  RTWFileNameOpts=Auto
  ~gb_trq_in_r : Product  Inputs=*//  Multiplication=Element-wise(.*)  SaturateOnIntegerOverflow=on
  "gear number, out" : Outport  Port=1  InitialOutput=0
  "gear ratio, out" : Outport  Port=2  InitialOutput=0
  "shifting, out" : Outport  Port=3  InitialOutput=0
  wires:
  Switch3/1 -> "gear number, out"/1
  Demux/2 -> "shifting, out"/1
  Demux/1 -> "gear ratio, out"/1
  Speed Dependent Shifting/2 -> [spd_dep_gear_num]
  Speed Dependent Shifting/1 -> [spd_dep_muxed]
  [v_req_limited] -> Speed Dependent Shifting/1
  [spd_dep_gear_num] -> Switch3/1
  Switch4/1 -> Demux/1
  [def_shifting] -> Mux/2
  [def_gear_ratio] -> Mux/1
  Mux/1 -> Switch4/3
  [spd_dep_muxed] -> Switch4/1
  Constant15/1 -> Switch4/2
  [def_gear_num] -> Switch3/3
  Constant14/1 -> Switch3/2
  gearbox speed estimator/1(Out1) -> To WS/1, downshift  command/3(engine speed), upshift  command/3(engine speed), engine torque capability/1
  allow upshift?/1(allow shift) -> Switch2/2
  upshift  command/1(command) -> Switch2/1
  Switch/1 -> downshift  command/2(engine load), upshift  command/2(engine load)
  Constant/1 -> Switch/1
  tires are at traction limit/1 -> Switch/2
  ~gb_trq_in_r/1 -> Product2/1
  Product2/1 -> load=T/ (maxT at spd)/1
  Rate Limiter/1 -> gear ratio/1
  gear ratio/1 -> prev gear ratio/1
  prev gear ratio/1 -> gb_spd_in_r/2, ~gb_trq_in_r/3
  gb_trq_out_r/1 -> ~gb_trq_in_r/1, allow upshift?/2(gb_trq_out_r)
  gb_spd_out_r/1 -> gb_spd_in_r/1, allow upshift?/3(gb_spd_out_r)
  Gain1/1 -> Switch1/1
  Constant2/1 -> Switch1/3
  Saturation/1 -> ~gb_trq_in_r/2, allow upshift?/4(prev Pout/Pin)
  prev. Pout/Pin/1 -> Saturation/1
  Constant1/1 -> Switch2/3
  prev gear number/1 -> current gear number/1, upshift  command/1(prev gear number), downshift  command/1(prev gear number), allow upshift?/1(prev gearnum), allow downshift?/1(prev gearnum)
  gear ratio1/1 -> [def_gear_ratio]
  Saturation1/1 -> [def_gear_num], Rate Limiter/1, shifting1/1(gear number), gear ratio1/1, prev gear number/1
  current gear number/1 -> Saturation1/1
  delta gear number/1 -> current gear number/2
  shifting1/1(out_1) -> [def_shifting]
  Switch2/1 -> delta gear number/1, delta gear number/2
  Switch1/1 -> delta gear number/3
  engine torque capability/1 -> Product2/2
  downshift  command/1(command) -> Gain1/1
  allow downshift?/1(allow shift) -> Switch1/2
  load=T/ (maxT at spd)/1 -> Switch/3
  gb_spd_in_r/1 -> gearbox speed estimator/1(gb_spd_in_r if no gear change)

== system BD_PAR_saber_cosim/Parallel Cosimulation/Model Data In ==
  Aux Loads 14V and 42V : Subsystem
      settings: RTWFcnNameOpts=Auto  RTWFileNameOpts=Auto
  DC/DC converter : lib_cosimulation/DC//DC converter
      settings: RTWFcnNameOpts=Auto  RTWFileNameOpts=Auto
  Matrix Concatenation1 : S-Function  FunctionName=smatrxcat  Parameters=numInports,catMethod  PortCounts=[]  SFunctionModules=''  mask(Matrix Concatenation){numInports=6, catMethod=Horizontal}
      mask prompts: numInports "Number of inputs:"; catMethod "Concatenation method:"
      mask help: Perform horizontal or vertical concatenation. 1-D vector input signals are treated as column vectors, i.e., [Mx1] matrices. The output is always a matrix.
      mask init:
      | xy = matrxcatmask('icon');
      mask StyleString: edit,popup(Horizontal|Vertical)
      mask Display:
      | plot(xy.x,xy.y);
      | text(0.15,0.86,xy.label);
  Regulator : lib_cosimulation/Regulator
      settings: RTWFcnNameOpts=Auto  RTWFileNameOpts=Auto
  ess param inputs : Subsystem  BlockChoice=Saber lib pb
      settings: AttributesFormatString=%<BlockChoice>  TemplateBlock=lib_cosimulation/ess param inputs  MemberBlocks=Rint,Saber lib pb  RTWFcnNameOpts=Auto  RTWFileNameOpts=Auto
  ess2 param inputs : Subsystem  BlockChoice=Saber lib pb2
      settings: AttributesFormatString=%<BlockChoice>  TemplateBlock=lib_cosimulation/ess2 param inputs  MemberBlocks=Rint2,Saber lib pb2  RTWFcnNameOpts=Auto  RTWFileNameOpts=Auto
  motor : lib_cosimulation/motor
      settings: RTWFcnNameOpts=Auto  RTWFileNameOpts=Auto
  Out1 : Outport  Port=1
  wires:
  ess2 param inputs/1(Out1) -> Matrix Concatenation1/4
  ess param inputs/1(Out1) -> Matrix Concatenation1/3
  Matrix Concatenation1/1 -> Out1/1
  Aux Loads 14V and 42V/1(Out1) -> Matrix Concatenation1/1
  DC/DC converter/1 -> Matrix Concatenation1/2
  Regulator/1 -> Matrix Concatenation1/5
  motor/1 -> Matrix Concatenation1/6

== system BD_PAR_saber_cosim/Parallel Cosimulation/Motor RPM Req ==
  w_apu : Inport  Port=1  LatchInput=off
  Constant : Constant  Value=0
  Enabled Subsystem : Subsystem  TreatAsAtomicUnit=on
      settings: RTWFcnNameOpts=Auto  RTWFileNameOpts=Auto
  IC : InitialCondition  Value=time_step
  Matrix Concatenation1 : S-Function  FunctionName=smatrxcat  Parameters=numInports,catMethod  PortCounts=[]  SFunctionModules=''  mask(Matrix Concatenation){numInports=6, catMethod=Horizontal}
      mask prompts: numInports "Number of inputs:"; catMethod "Concatenation method:"
      mask help: Perform horizontal or vertical concatenation. 1-D vector input signals are treated as column vectors, i.e., [Mx1] matrices. The output is always a matrix.
      mask init:
      | xy = matrxcatmask('icon');
      mask StyleString: edit,popup(Horizontal|Vertical)
      mask Display:
      | plot(xy.x,xy.y);
      | text(0.15,0.86,xy.label);
  Memory1 : Memory  X0=.001  InheritSampleTime=on
      settings: RTWStateStorageClass=Auto
  Memory2 : Memory  X0=0  InheritSampleTime=on
      settings: RTWStateStorageClass=Auto
  Relational Operator : RelationalOperator  Operator===
  Saturation : Saturate  UpperLimit=inf  LowerLimit=.001  LinearizeAsGain=on
  mc_rpm_r : Scope
      settings: TimeRange=10  YMin=0  YMax=2000  SaveToWorkspace=off  SaveName=ScopeData5  LimitDataPoints=on  MaxDataPoints=5000
  "rad/s -> rpm1" : Gain  Gain=60/(2*pi)  Multiplication=Element-wise(K.*u)  SaturateOnIntegerOverflow=on
  RPM : Outport  Port=1
  wires:
  Relational Operator/1 -> Enabled Subsystem/Enable
  [time] -> Relational Operator/2
  Enabled Subsystem/1(Out1) -> Matrix Concatenation1/2
  Memory2/1 -> Matrix Concatenation1/4
  Matrix Concatenation1/1 -> RPM/1
  IC/1 -> Matrix Concatenation1/5
  Saturation/1 -> Memory1/1
  [time] -> Saturation/1
  Memory1/1 -> Matrix Concatenation1/3
  [time] -> IC/1
  Constant/1 -> Relational Operator/1, Matrix Concatenation1/1
  w_apu/1 -> "rad/s -> rpm1"/1
  "rad/s -> rpm1"/1 -> Memory2/1, Matrix Concatenation1/6, mc_rpm_r/1, Enabled Subsystem/1(In1)

== system BD_PAR_saber_cosim/Parallel Cosimulation/Motor Trq Req ==
  trq : Inport  Port=1  LatchInput=off
  Constant : Constant  Value=0
  Enabled Subsystem : Subsystem  TreatAsAtomicUnit=on
      settings: RTWFcnNameOpts=Auto  RTWFileNameOpts=Auto
  IC : InitialCondition  Value=time_step
  Matrix Concatenation2 : S-Function  FunctionName=smatrxcat  Parameters=numInports,catMethod  PortCounts=[]  SFunctionModules=''  mask(Matrix Concatenation){numInports=6, catMethod=Horizontal}
      mask prompts: numInports "Number of inputs:"; catMethod "Concatenation method:"
      mask help: Perform horizontal or vertical concatenation. 1-D vector input signals are treated as column vectors, i.e., [Mx1] matrices. The output is always a matrix.
      mask init:
      | xy = matrxcatmask('icon');
      mask StyleString: edit,popup(Horizontal|Vertical)
      mask Display:
      | plot(xy.x,xy.y);
      | text(0.15,0.86,xy.label);
  Memory1 : Memory  X0=.001  InheritSampleTime=on
      settings: RTWStateStorageClass=Auto
  Memory2 : Memory  X0=0  InheritSampleTime=on
      settings: RTWStateStorageClass=Auto
  Relational Operator : RelationalOperator  Operator===
  Saturation : Saturate  UpperLimit=inf  LowerLimit=.001  LinearizeAsGain=on
  mc_trq_r : Scope
      settings: TimeRange=10  YMin=0  YMax=600  SaveToWorkspace=off  SaveName=ScopeData4  LimitDataPoints=on  MaxDataPoints=5000
  trq array : Outport  Port=1
  wires:
  trq/1 -> Enabled Subsystem/1(In1), Memory2/1, Matrix Concatenation2/6, mc_trq_r/1
  Constant/1 -> Matrix Concatenation2/1, Relational Operator/1
  [time] -> IC/1
  Memory1/1 -> Matrix Concatenation2/3
  [time] -> Saturation/1
  Saturation/1 -> Memory1/1
  IC/1 -> Matrix Concatenation2/5
  Matrix Concatenation2/1 -> trq array/1
  Memory2/1 -> Matrix Concatenation2/4
  Enabled Subsystem/1(Out1) -> Matrix Concatenation2/2
  [time] -> Relational Operator/2
  Relational Operator/1 -> Enabled Subsystem/Enable

== system BD_PAR_saber_cosim/Parallel Cosimulation/Parallel Cosim ==
  In : Inport  Port=1  LatchInput=off
  Par Saber Text File Exchange : lib_cosimulation/Par Saber Text File Exchange
  out : Outport  Port=1
  wires:
  In/1 -> Par Saber Text File Exchange/1
  Par Saber Text File Exchange/1 -> out/1

== system BD_PAR_saber_cosim/Parallel Cosimulation/Saber_ess2_outputs ==
  In1 : Inport  Port=1  LatchInput=off
  Saber_pb2 : lib_outputs/Saber_pb2
      settings: RTWFcnNameOpts=Auto  RTWFileNameOpts=Auto
  wires:
  In1/1 -> Saber_pb2/1

== system BD_PAR_saber_cosim/Parallel Cosimulation/Saber_ess_outputs ==
  In1 : Inport  Port=1  LatchInput=off
  Saber_pb : lib_outputs/Saber_pb
      settings: RTWFcnNameOpts=Auto  RTWFileNameOpts=Auto
  wires:
  In1/1 -> Saber_pb/1

== system BD_PAR_saber_cosim/Parallel Cosimulation/if trq_req <=1 trq_ach = trq_req & spd_ach=spd_req ==
  ach : Inport  Port=1  LatchInput=off
  req : Inport  Port=2  LatchInput=off
  Abs : Abs  SaturateOnIntegerOverflow=on
  Constant : Constant  Value=1
  Relational Operator : RelationalOperator  Operator=<=
  Switch : Switch  Threshold=eps
  trq r : Selector  InputType=Vector  ElementSrc=Internal  Elements=[1]  RowSrc=Internal  Rows=1  ColumnSrc=Internal  Columns=1  InputPortWidth=2
  Out1 : Outport  Port=1
  wires:
  req/1 -> trq r/1, Switch/1
  Switch/1 -> Out1/1
  Relational Operator/1 -> Switch/2
  Constant/1 -> Relational Operator/2
  Abs/1 -> Relational Operator/1
  ach/1 -> Switch/3
  trq r/1 -> Abs/1

== system BD_PAR_saber_cosim/<vc> par/engine on (parallel hybrid)/Block NOTES1 ==
  note: This engine state computer keeps the engine on if:
      | [
      | 1) key is on, AND
      | 2) (trq is too high AND speed is too high for idle) OR engine is allowed to idle, AND
      | 3) vehicle speed >= cs_electric_launch_spd [ in m/s ], AND
      | 4) req'd trq > (cs_off_trq_frac * max_trq_at_spd) OR SOC<cs_lo_soc
      | ]
      | OR
      | [ engine was previously on AND the transmission is shifting ]
      |
      | The last condition is added to prevent the engine from unrealistically
      | shutting down for a second or two during a shift.

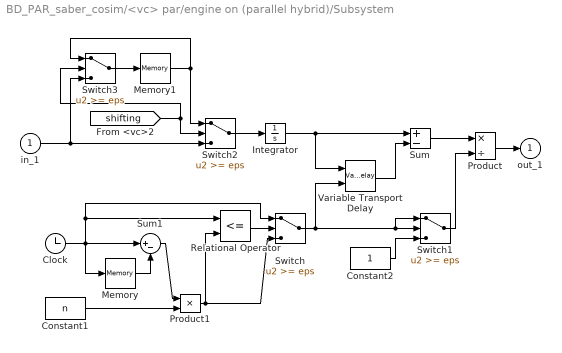
== system BD_PAR_saber_cosim/<vc> par/engine on (parallel hybrid)/Subsystem ==
  in_1 : Inport  Port=1  LatchInput=off
  Clock : Clock
      settings: DisplayTime=off  Decimation=10
  Constant1 : Constant  Value=n
  Constant2 : Constant  Value=1
  Integrator : Integrator  ExternalReset=none  InitialConditionSource=internal  InitialCondition=0  LimitOutput=off  UpperSaturationLimit=inf  LowerSaturationLimit=-inf  ShowSaturationPort=off  ShowStatePort=off  AbsoluteTolerance=auto
  Memory : Memory  X0=-0.1  InheritSampleTime=off
      settings: RTWStateStorageClass=Auto
  Memory1 : Memory  X0=0  InheritSampleTime=off
      settings: RTWStateStorageClass=Auto
  Product : Product  Inputs=*/  Multiplication=Element-wise(.*)  SaturateOnIntegerOverflow=on
  Product1 : Product  Inputs=2  Multiplication=Element-wise(.*)  SaturateOnIntegerOverflow=on
  Relational Operator : RelationalOperator  Operator=<=
  Sum : Sum  Inputs=+-  SaturateOnIntegerOverflow=on
  Sum1 : Sum  Inputs=|+-  SaturateOnIntegerOverflow=on
  Switch{,1..3} (4 alike) : Switch  Threshold=eps
  Variable Transport Delay : VariableTransportDelay  MaximumDelay=n  InitialInput=0  MaximumPoints=1024  PadeOrder=0
  out_1 : Outport  Port=1  InitialOutput=0
  wires:
  Product/1 -> out_1/1
  Sum/1 -> Product/1
  Variable Transport Delay/1 -> Sum/2
  Integrator/1 -> Variable Transport Delay/1, Sum/1
  Relational Operator/1 -> Switch/2
  Constant1/1 -> Product1/2
  Clock/1 -> Sum1/1, Memory/1, Relational Operator/1, Switch/1
  Memory/1 -> Sum1/2
  Sum1/1 -> Product1/1
  Product1/1 -> Relational Operator/2, Switch/3
  Switch/1 -> Variable Transport Delay/2, Switch1/2, Switch1/1
  Constant2/1 -> Switch1/3
  Switch1/1 -> Product/2
  Switch2/1 -> Integrator/1
  Switch3/1 -> Memory1/1
  in_1/1 -> Switch2/3, Switch3/3
  Memory1/1 -> Switch2/1, Switch3/1
  [shifting] -> Switch2/2, Switch3/2

== system BD_PAR_saber_cosim/<vc> par/engine on (parallel hybrid)/key_on ==
  Clock : Clock
      settings: DisplayTime=off  Decimation=10
  Fcn1 : Fcn  Expr=rem(u[1],period)
  Look-Up Table : Lookup  InputValues=t  OutputValues=y
  out_1 : Outport  Port=1  InitialOutput=0
  wires:
  Fcn1/1 -> Look-Up Table/1
  Clock/1 -> Fcn1/1
  Look-Up Table/1 -> out_1/1

== system BD_PAR_saber_cosim/<vc> par/engine on (parallel hybrid)/repeated cycle:  speed required at end of NEXT step ==
  Clock : Clock
      settings: DisplayTime=off  Decimation=10
  Fcn1 : Fcn  Expr=rem(u[1],period)
  Look-Up Table : Lookup  InputValues=t  OutputValues=y
  Memory : Memory  X0=-0.1  InheritSampleTime=off
      settings: RTWStateStorageClass=Auto
  Sum : Sum  Inputs=+-  SaturateOnIntegerOverflow=on
  Sum1 : Sum  Inputs=++  SaturateOnIntegerOverflow=on
  out_1 : Outport  Port=1  InitialOutput=0
  wires:
  Sum1/1 -> Look-Up Table/1
  Look-Up Table/1 -> out_1/1
  Fcn1/1 -> Sum1/1
  Sum/1 -> Sum1/2
  Memory/1 -> Sum/2
  Clock/1 -> Fcn1/1, Memory/1, Sum/1
